simulink model "pid_sim"  (R2024b)
settings: Solver=ode15s  StartTime=0.0  StopTime=simTime  FixedStep=0.1  MaxStep=0.01  RelTol=1e-3  AbsTol=1e-6
undefined symbols (not defined in the file): A, C, kd, ki, kp, setpoint
settings Model: PacingRate=100  Creator=SeniyaMinsikaWeeraso  LastModifiedBy=labadmin

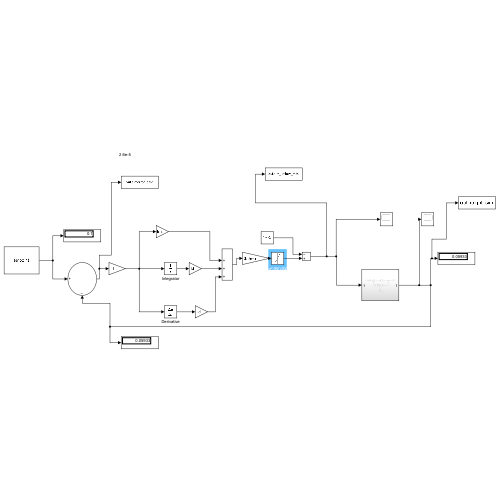
[thumbnail: Simulink's stored preview of the top-level diagram]
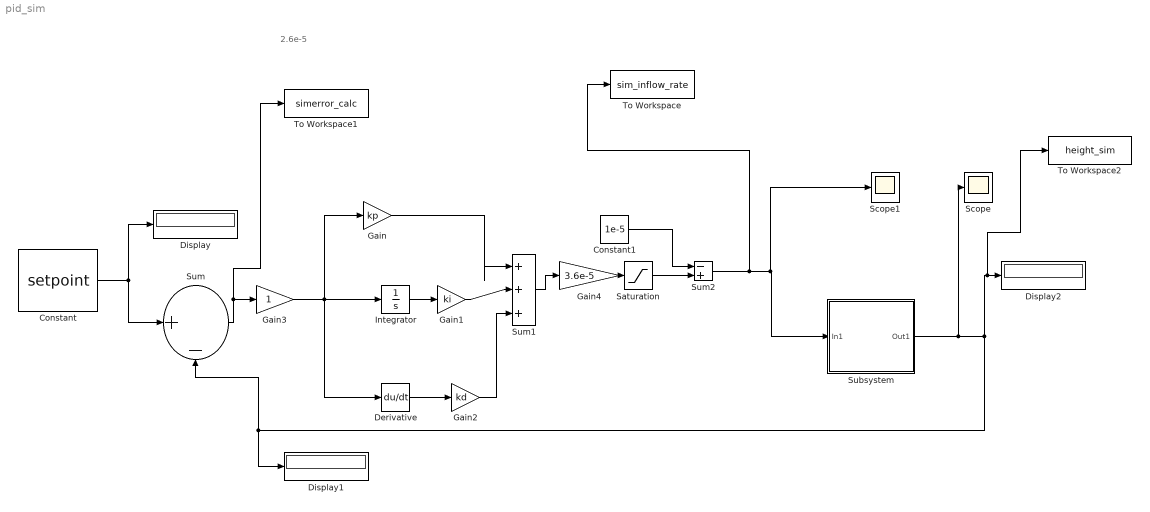
== system pid_sim ==
  note: 2.6e-5
  Constant : Constant  Value=setpoint
  Constant1 : Constant  Value=1e-5
  Derivative : Derivative
  Display : Display
  Display1 : Display
  Display2 : Display
  Gain : Gain  Gain=kp
  Gain1 : Gain  Gain=ki
  Gain2 : Gain  Gain=kd
  Gain3 : Gain
  Gain4 : Gain  Gain=3.6e-5
  Integrator : Integrator
  Saturation : Saturate  UpperLimit=3.6e-5  LowerLimit=1e-5
  Scope : Scope
  Scope1 : Scope
  Subsystem : Subsystem
  Sum : Sum  Inputs=|+-
  Sum1 : Sum  Inputs=|+++
  Sum2 : Sum  Inputs=-+
  To Workspace : ToWorkspace  VariableName=sim_inflow_rate  SaveFormat=Structure With Time  SampleTime=-1
  To Workspace1 : ToWorkspace  VariableName=simerror_calc  SaveFormat=Structure With Time  SampleTime=-1
  To Workspace2 : ToWorkspace  VariableName=height_sim  SaveFormat=Structure With Time  SampleTime=-1
  wires:
  Subsystem/1(Out1) -> Scope/1, To Workspace2/1, Display2/1, Sum/2, Display1/1
  Constant/1 -> Display/1, Sum/1
  Sum/1 -> To Workspace1/1, Gain3/1
  Gain/1 -> Sum1/1
  Gain1/1 -> Sum1/2
  Gain2/1 -> Sum1/3
  Integrator/1 -> Gain1/1
  Derivative/1 -> Gain2/1
  Gain3/1 -> Derivative/1, Gain/1, Integrator/1
  Sum1/1 -> Gain4/1
  Gain4/1 -> Saturation/1
  Sum2/1 -> To Workspace/1, Scope1/1, Subsystem/1(In1)
  Constant1/1 -> Sum2/1
  Saturation/1 -> Sum2/2

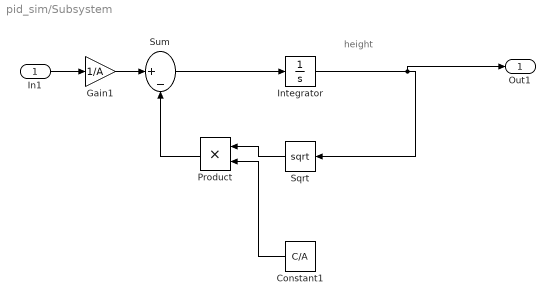
== system pid_sim/Subsystem ==
  note: height
  In1 : Inport
  Constant1 : Constant  Value=C/A
  Gain1 : Gain  Gain=1/A
  Integrator : Integrator
  Product : Product
  Sqrt : Sqrt
  Sum : Sum  Inputs=|+-
  Out1 : Outport
  wires:
  Integrator/1 -> Out1/1, Sqrt/1
  In1/1 -> Gain1/1
  Gain1/1 -> Sum/1
  Sum/1 -> Integrator/1
  Product/1 -> Sum/2
  Sqrt/1 -> Product/1
  Constant1/1 -> Product/2
